simulink model "FIRP_nl"  (R2020a)
settings: Solver=FixedStepAuto  StartTime=0.0  StopTime=time  FixedStep=0.05  RelTol=1e-5
InitFcn:
  | variableCalc
values from neighbouring files (symbols this model uses):
  aD1 = 10    [variableCalc.m]
  bd = zeros(3,1)    [variableCalc.m]
  cd = [0 1 0; 0 0 1]    [variableCalc.m]
  d0 = [aD1;0;aD2]    [variableCalc.m]
  dd = [0;0]    [variableCalc.m]
  S = [0 0 0 ... (first row only)    [variableCalc.m]
  wD1 = 10    [variableCalc.m]
  x0 = [0;1;0;0.7]    [variableCalc.m]
settings Model: Creator=alfystar  LastModifiedBy=emanu

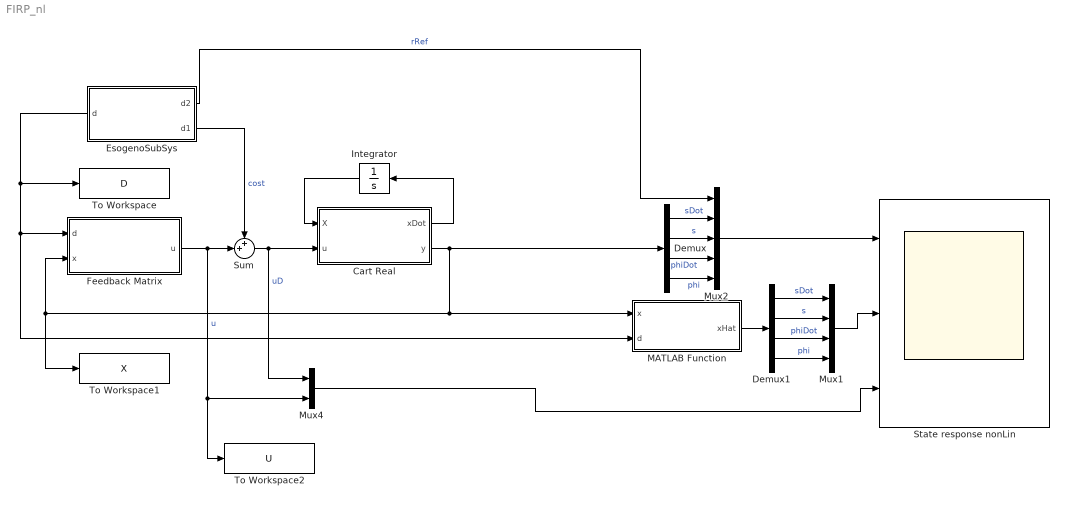
== system FIRP_nl ==
  Cart Real : MATLAB Function  TreatAsAtomicUnit=on
  Demux : Demux
  Demux1 : Demux
  EsogenoSubSys : Subsystem
      settings: PortSchema="{\"entries\":[{\"content\":{\"sides\":[{\"content\":{\"connectorIds\":[\"Out3\"]},\"type\":\"ConnectorPlacement.EquallySpacedRectSide\",\"uuid\":\"2f048b8f-2ece-4481-a059-706f1c660597\"},{\"content\":{\"connectorIds\":[\"Out1\",\"Out2\"],\"side\":\"RIGHT\"},\"type\":\"ConnectorPlacement.EquallySpacedRectSide\",\"uuid\":\"5f2d4447-8f06-4961-a5d4-88bfa1a982d6\"},{\"content\":{\"connectorIds\":[],\"side\":\"TOP\"},\"type\":\"ConnectorPlacement.EquallySpacedRectSide\",\"uuid\":\"01607c17-a512-406e-96e4-6df13fd083f1\"}]},\"type\":\"ConnectorPlacement.EquallySpacedConnector\",\"uuid\":\"68a4d915-b1c1-450a-8606-a9ee066c43ba\"}],\"packageUris\":[\"http://schema.mathworks.com/mf0/Connector/19700101\"],\"version\":\"1.0\"}"
  Feedback Matrix : MATLAB Function  TreatAsAtomicUnit=on
  Integrator : Integrator  InitialCondition=x0
  MATLAB Function : MATLAB Function  TreatAsAtomicUnit=on
  Mux1 : Mux
  Mux2 : Mux  Inputs=5
  Mux4 : Mux  Inputs=2
  State response nonLin : Scope  NumInputPorts=3
  Sum : Sum  Inputs=++|
  To Workspace : ToWorkspace  VariableName=D  SaveFormat=Timeseries  SampleTime=-1
  To Workspace1 : ToWorkspace  VariableName=X  SaveFormat=Timeseries  SampleTime=-1
  To Workspace2 : ToWorkspace  VariableName=U  SaveFormat=Timeseries  SampleTime=-1
  wires:
  Cart Real/2(y) -> Demux/1, To Workspace1/1, Feedback Matrix/2(x), MATLAB Function/1(x)
  Demux/3 -> Mux2/4  "phiDot"
  Demux/4 -> Mux2/5  "phi"
  Mux2/1 -> State response nonLin/1
  Feedback Matrix/1(u) -> To Workspace2/1, Mux4/2, Sum/2  "u"
  Demux/1 -> Mux2/2  "sDot"
  Demux/2 -> Mux2/3  "s"
  Sum/1 -> Cart Real/2(u), Mux4/1  "uD"
  Mux4/1 -> State response nonLin/3
  EsogenoSubSys/3(d) -> To Workspace/1, Feedback Matrix/1(d), MATLAB Function/2(d)
  EsogenoSubSys/2(d1) -> Sum/1  "cost"
  EsogenoSubSys/1(d2) -> Mux2/1  "rRef"
  Demux1/3 -> Mux1/3  "phiDot"
  Demux1/4 -> Mux1/4  "phi"
  Demux1/2 -> Mux1/2  "s"
  MATLAB Function/1(xHat) -> Demux1/1
  Demux1/1 -> Mux1/1  "sDot"
  Mux1/1 -> State response nonLin/2
  Cart Real/1(xDot) -> Integrator/1
  Integrator/1 -> Cart Real/1(X)

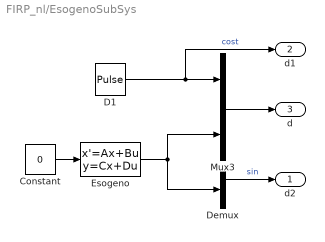
== system FIRP_nl/EsogenoSubSys ==
  Constant : Constant  Value=0
  D1 : DiscretePulseGenerator  PulseType=Time based  Amplitude=aD1  Period=wD1  PulseWidth=50
  Demux : Demux  Outputs=2
  Esogeno : StateSpace  A=S  B=bd  C=cd  D=dd  InitialCondition=d0
  Mux3 : Mux  Inputs=2
  d2 : Outport
  d1 : Outport  Port=2
  d : Outport  Port=3
  wires:
  D1/1 -> d1/1, Mux3/1  "cost"
  Esogeno/1 -> Demux/1, Mux3/2
  Constant/1 -> Esogeno/1
  Mux3/1 -> d/1
  Demux/1 -> d2/1  "sin"

== matlab function FIRP_nl/MATLAB Function ==
  data: x input; xHat output; d input
function xHat = baseChange(x,d)

coder.extrinsic('evalin', 'assignin')
PiMat = zeros(4,3);                  % Needed in order to set variable class correctly
PiMat = evalin('base','PiMat'); % Read value from workspace


xHat = x-PiMat*d;
end

== matlab function FIRP_nl/Feedback Matrix ==
  data: d input; x input; u output
function u = feedMatrix(d,x)

coder.extrinsic('evalin', 'assignin')
K = zeros(1,4);                  % Needed in order to set variable class correctly
K = evalin('base','K'); % Read value from workspace

L = zeros(1,3);                  % Needed in order to set variable class correctly
L = evalin('base','L'); % Read value from workspace

% x(2)=x(2)-d(2);
u = 0;
u = K*x+L*d;
end

== matlab function FIRP_nl/Cart Real ==
  data: xDot output; X input; u input; y output
function [xDot,y] = CartSis(X,u)

coder.extrinsic('evalin', 'assignin')
l=1;
l = evalin('base','l'); % Read value from workspace

M=1;
M = evalin('base','M'); % Read value from workspace

F=1;
F = evalin('base','F'); % Read value from workspace

g=9.81;
g = evalin('base','g'); % Read value from workspace

y=X;

xDot=zeros(4,1);
xDot(1) = (u - F*X(1))/M;
xDot(2) = X(1);
xDot(3) = g/l*sin(X(4))+(xDot(1)/l)*cos(X(4));

xDot(4) = X(3);
% xDot
% y

end
